simulink model "EKF_unknown"  (R2020b)
settings: Solver=ode45  StartTime=0.0  StopTime=50  FixedStep=1e-7  RelTol=1e-4  AbsTol=1e-4  EnableMultiTasking=on
libraries: simulink x1
settings Model: EnablePacing=on  PacingRate=10  Creator=André  LastModifiedBy=Andre
settings SolverCC: AutoScaleAbsTol=off  ConsecutiveZCsStepRelTol=100*128*eps  ShapePreserveControl=EnableAll  ZeroCrossControl=EnableAll  AutoInsertRateTranBlk=on
settings DataIOCC: LimitDataPoints=on  SaveFormat=Array  SignalLoggingSaveFormat=ModelDataLogs  ReturnWorkspaceOutputs=off
settings OptimizationCC: ExpressionDepthLimit=2147483647  LifeSpan=inf
settings DebuggingCC: UnderspecifiedInitializationDetection=Classic  MergeDetectMultiDrivingBlocksExec=none  SolverPrmCheckMsg=warning  FcnCallInpInsideContextMsg=warning  StateNameClashWarn=warning  SFUnexpectedBacktrackingDiag=warning  SFNoUnconditionalDefaultTransitionDiag=warning  SFExecutionAtInitializationDiag=none  ArithmeticOperatorsInVariantConditions=warning
settings HardwareCC: ProdBitPerPointer=32  ProdBitPerSizeT=32  ProdBitPerPtrDiffT=32  ProdLargestAtomicFloat=None  ProdIntDivRoundTo=Undefined  ProdEndianess=Unspecified  ProdWordSize=32  ProdHWDeviceType=32-bit Generic
settings ModelReferenceCC: PropagateSignalLabelsOutOfModel=off
settings SFSimCC: SimUseLocalCustomCode=off  SimParseCustomCode=off  CustomCodeUndefinedFunction=UseInterfaceOnly
settings RTWCC: RTWUseLocalCustomCode=off
settings CodeAppCC: StateflowObjectComments=on
settings GRTTargetCC: TargetLangStandard=C89/C90 (ANSI)  CombineOutputUpdateFcns=off  GRTInterface=on
settings ConfigComp: CovMetricSettings=dw  CovSaveCumulativeToWorkspaceVar=on  CovSaveSingleToWorkspaceVar=on  CovExternalEMLEnable=off

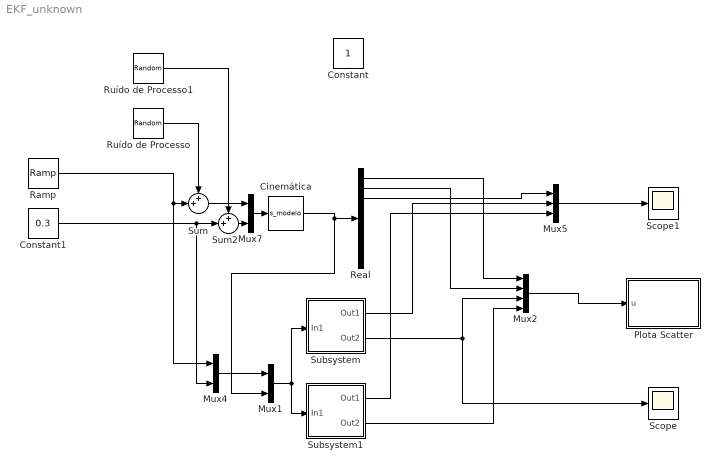
== system EKF_unknown ==
  Cinemática : S-Function  FunctionName=s_modelo  Parameters=[0 -5 -pi/4]  SFunctionDeploymentMode=off  EnableBusSupport=off
  Constant : Constant
  Constant1 : Constant  Value=0.3
  Mux1 : Mux  Inputs=2
  Mux2 : Mux
  Mux4 : Mux  Inputs=2
  Mux5 : Mux  Inputs=3
  Mux7 : Mux  Inputs=2
  Plota Scatter : MATLAB Function  TreatAsAtomicUnit=on  SystemSampleTime=0.5
  Ramp : simulink/Sources/Ramp  slope=0.05  start=0  InitialOutput=1
  Real : Demux  Outputs=9
  Ruído de Processo : RandomNumber  Variance=0.1  SampleTime=0.1
  Ruído de Processo1 : RandomNumber  Variance=0.1  SampleTime=0.1
  Scope : Scope
  Scope1 : Scope
  Subsystem : Subsystem
  Subsystem1 : Subsystem
  Sum : Sum  Inputs=++|
  Sum2 : Sum  Inputs=++|
  wires:
  Ruído de Processo/1 -> Sum/1
  Mux7/1 -> Cinemática/1
  Sum2/1 -> Mux7/2
  Ramp/1 -> Mux4/1, Sum/2
  Sum/1 -> Mux7/1
  Mux4/1 -> Mux1/1
  Cinemática/1 -> Mux1/2, Real/1
  Constant1/1 -> Mux4/2, Sum2/2
  Ruído de Processo1/1 -> Sum2/1
  Real/1 -> Mux2/1
  Real/2 -> Mux2/2
  Mux2/1 -> Plota Scatter/1(u)
  Real/3 -> Mux5/1
  Mux5/1 -> Scope1/1
  Subsystem/2(Out2) -> Scope/1, Mux2/3
  Mux1/1 -> Subsystem/1(In1), Subsystem1/1(In1)
  Subsystem/1(Out1) -> Mux5/2
  Subsystem1/1(Out1) -> Mux5/3
  Subsystem1/2(Out2) -> Mux2/4

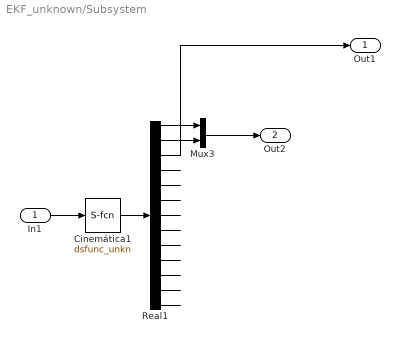
== system EKF_unknown/Subsystem ==
  In1 : Inport
  Cinemática1 : S-Function  FunctionName=dsfunc_unkn  Parameters=[-5 5 0 10 0 0 0 10 0 0 0 10 0]  SFunctionDeploymentMode=off  EnableBusSupport=off
  Mux3 : Mux  Inputs=2
  Real1 : Demux  Outputs=13
  Out1 : Outport
  Out2 : Outport  Port=2
  wires:
  Real1/3 -> Out1/1
  Real1/10 -> ?
  Real1/7 -> ?
  Cinemática1/1 -> Real1/1
  Real1/13 -> ?
  Mux3/1 -> Out2/1
  Real1/1 -> Mux3/1
  Real1/2 -> Mux3/2
  In1/1 -> Cinemática1/1
  Real1/12 -> ?
  Real1/11 -> ?
  Real1/4 -> ?
  Real1/8 -> ?
  Real1/5 -> ?
  Real1/6 -> ?
  Real1/9 -> ?

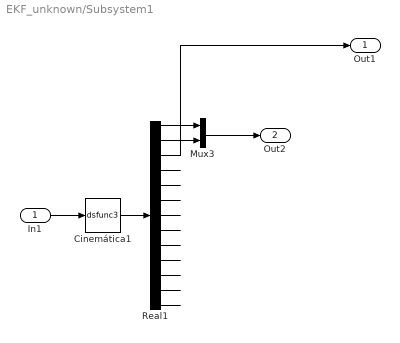
== system EKF_unknown/Subsystem1 ==
  In1 : Inport
  Cinemática1 : S-Function  FunctionName=dsfunc3  Parameters=[-5 5 0 10 0 0 0 10 0 0 0 10 0]  SFunctionDeploymentMode=off  EnableBusSupport=off
  Mux3 : Mux  Inputs=2
  Real1 : Demux  Outputs=13
  Out1 : Outport
  Out2 : Outport  Port=2
  wires:
  Real1/3 -> Out1/1
  Real1/10 -> ?
  Real1/7 -> ?
  Cinemática1/1 -> Real1/1
  Real1/13 -> ?
  Mux3/1 -> Out2/1
  Real1/1 -> Mux3/1
  Real1/2 -> Mux3/2
  In1/1 -> Cinemática1/1
  Real1/12 -> ?
  Real1/11 -> ?
  Real1/4 -> ?
  Real1/8 -> ?
  Real1/5 -> ?
  Real1/6 -> ?
  Real1/9 -> ?

== matlab function EKF_unknown/Plota Scatter ==
  data: u input
function  fcn(u)
     %n_Particulas = 1000;  
    marker = [0 -5; 0 5]; % Positions of markers
    ax =[-20 20 -20 20];
     %n_estados = n_Particulas*3;
     x = u(1:2);
     xx = u(3:4);
     xxx= u(5:6);
     %particulas = u(3:(2+n_estados));
     coder.extrinsic('scatter')
     coder.extrinsic('subplot')
     
      %xP = reshape(particulas,3,[]);
      %x_ = mean(xP, 2);
      %x_ = u(3+n_estados:5+n_estados);
      %scatter(xP(1,:),xP(2,:), 'k.');
      subplot(2,2,1)
      
      hold off;
      
      scatter(xx(1),xx(2),'bo');
      axis( ax);
      hold on
      scatter(marker(:,1),marker(:,2), 'ms','MarkerFaceColor','m');
      scatter(x(1),x(2), 'r*');
      hold off;
      
      subplot(2,2,2)
      
      hold off;
      scatter(xxx(1),xxx(2),'bo');
      axis( ax);
      hold on
      scatter(marker(1,1),marker(1,2), 'ms','MarkerFaceColor','b');
      scatter(marker(2,1),marker(2,2), 'ms','MarkerFaceColor','g');
      scatter(x(1),x(2), 'r*');
      hold off;
      
      
     subplot(2,2,3)
      
      hold on;
      
      scatter(xx(1),xx(2),'bo');
      axis( ax);
      hold on
      scatter(marker(:,1),marker(:,2), 'ms','MarkerFaceColor','m');
      scatter(x(1),x(2), 'r*');
      hold off;
      
      subplot(2,2,4)
      
      hold on;
      scatter(xxx(1),xxx(2),'bo');
      axis( ax);
      hold on
      scatter(marker(1,1),marker(1,2), 'ms','MarkerFaceColor','b');
      scatter(marker(2,1),marker(2,2), 'ms','MarkerFaceColor','g');
      scatter(x(1),x(2), 'r*');
      hold off;
     % insert additional code as needed to turn on grid, setup axis limits, etc.

  %%%%%%%%%
%y = u;
